simulink library "cpcAux"  (R2016a)
settings: Solver=ode45  StartTime=0.0  StopTime=10.0  RelTol=1e-3
undefined symbols (not defined in the file): DiscIntNeverNeededParam, sMP
libraries: simulink x16, cpcAux x8
(part 2 of 2)

== system cpcAux/cpcAux/Other/motion detected ==
  u : Inport
  Compare : RelationalOperator  Operator=>  OutDataTypeStr=fixdt(0, 8)  ZeroCross=off  InputSameDT=on
  Constant : Constant  DisableCoverage=on  Value=const  OutDataTypeStr=Inherit: Inherit via back propagation
  y : Outport
  wires:
  Compare/1 -> y/1
  Constant/1 -> Compare/2
  u/1 -> Compare/1

== system cpcAux/cpcAux/Shift/round for Voith DIWA transmissions ==
  note: round to defined resolution
  In1 : Inport
  Constant : Constant  Value=1/resolution
      settings: AttributesFormatString=%<Value>
  Divide : Product  Inputs=*/
  Product : Product
  Rounding Function : Rounding  Operator=round
  Out1 : Outport
  wires:
  In1/1 -> Product/1
  Divide/1 -> Out1/1
  Rounding Function/1 -> Divide/1
  Product/1 -> Rounding Function/1
  Constant/1 -> Product/2, Divide/2

== system cpcAux/cpcAux/Shift/shift manually for eActros ==
  kmh : Inport
  gear : Inport  Port=2
  sw_in : Inport  Port=3
  Chart : Stateflow chart  TreatAsAtomicUnit=on
  Constant : Constant  Value=bShiftManual
  SNA CurrGr : Subsystem  mask{sna_max=129, sna_eq=0}
      mask prompts: sna_max "max value"; sna_eq "equivalent value"
      mask help: If value above max value, it will be replaced by equivalent value
      settings: AttributesFormatString=x > %<sna_max>: %<sna_eq>
  consider manual shift from driver : Switch  Criteria=u2 > Threshold
  manual shift from cpcAux : Switch  Criteria=u2 > Threshold
  no shift : simulink/Logic and Bit Operations/Compare To Constant  relop===  const=1  OutDataTypeStr=boolean
  sw_out : Outport
  wires:
  manual shift from cpcAux/1 -> sw_out/1
  Constant/1 -> manual shift from cpcAux/2
  gear/1 -> SNA CurrGr/1(In)
  consider manual shift from driver/1 -> manual shift from cpcAux/1
  no shift/1 -> consider manual shift from driver/2
  Chart/1(sw) -> consider manual shift from driver/1
  kmh/1 -> Chart/1(kmh)
  sw_in/1 -> no shift/1, consider manual shift from driver/3, manual shift from cpcAux/3
  SNA CurrGr/1(Out) -> Chart/2(gear)

== system cpcAux/cpcAux/eActros Drivertrain ready/PT Ready Check ==
  PT_ready : Inport
  Enable : EnablePort
  Constant : Constant
  Discrete-Time Integrator : DiscreteIntegrator  gainval=1  InitialConditionSetting=State (most efficient)  SampleTime=-1  ICPrevOutput=DiscIntNeverNeededParam  ICPrevScaledInput=DiscIntNeverNeededParam
  Logical Operator : Logic  Operator=OR  AllPortsSameDT=off  OutDataTypeStr=boolean
  Logical Operator1 : Logic  Operator=NOT  Inputs=1  AllPortsSameDT=off  OutDataTypeStr=boolean
  Stop__Powertrain_not_ready : Stop  Description=The simulation completes the current time step before terminating
      settings: AttributesFormatString=%<Description>
  affter 1min : simulink/Logic and Bit Operations/Compare To Constant  relop=<  const=60  OutDataTypeStr=boolean
  error_pt_ready : Assertion  AssertionFailFcn=fprintf(2,'cpcAux: PT not ready, even after 60s after ignition\n')  StopWhenAssertionFail=off
  wires:
  Logical Operator1/1 -> Stop__Powertrain_not_ready/1
  Logical Operator/1 -> error_pt_ready/1, Logical Operator1/1
  affter 1min/1 -> Logical Operator/1
  Discrete-Time Integrator/1 -> affter 1min/1
  Constant/1 -> Discrete-Time Integrator/1
  PT_ready/1 -> Logical Operator/2

== system cpcAux/cpcAux/CruiseControl/CC controlled by IPPC/Interval ==
  u : Inport
  AND : Logic  AllPortsSameDT=off  OutDataTypeStr=boolean
  FixPt Data Type Duplicate : DataTypeDuplicate  DisableCoverage=on  NumInputPorts=3
  Lower Limit : Constant  DisableCoverage=on  Value=lowlimit  OutDataTypeStr=Inherit: Inherit via back propagation
  Lower Test : RelationalOperator  DisableCoverage=on  Operator=<=  OutDataTypeStr=boolean  ZeroCross=off
  Upper Limit : Constant  DisableCoverage=on  Value=uplimit  OutDataTypeStr=Inherit: Inherit via back propagation
  Upper Test : RelationalOperator  DisableCoverage=on  Operator=<=  OutDataTypeStr=boolean  ZeroCross=off
  y : Outport
  wires:
  AND/1 -> y/1
  u/1 -> Upper Test/1, Lower Test/2, FixPt Data Type Duplicate/1
  Upper Test/1 -> AND/2
  Lower Test/1 -> AND/1
  Upper Limit/1 -> FixPt Data Type Duplicate/3, Upper Test/2
  Lower Limit/1 -> FixPt Data Type Duplicate/2, Lower Test/1

== system cpcAux/cpcAux/CruiseControl/CC controlled by IPPC/Interval1 ==
  u : Inport
  AND : Logic  AllPortsSameDT=off  OutDataTypeStr=boolean
  FixPt Data Type Duplicate : DataTypeDuplicate  DisableCoverage=on  NumInputPorts=3
  Lower Limit : Constant  DisableCoverage=on  Value=lowlimit  OutDataTypeStr=Inherit: Inherit via back propagation
  Lower Test : RelationalOperator  DisableCoverage=on  Operator=<=  OutDataTypeStr=boolean  ZeroCross=off
  Upper Limit : Constant  DisableCoverage=on  Value=uplimit  OutDataTypeStr=Inherit: Inherit via back propagation
  Upper Test : RelationalOperator  DisableCoverage=on  Operator=<=  OutDataTypeStr=boolean  ZeroCross=off
  y : Outport
  wires:
  AND/1 -> y/1
  u/1 -> Upper Test/1, Lower Test/2, FixPt Data Type Duplicate/1
  Upper Test/1 -> AND/2
  Lower Test/1 -> AND/1
  Upper Limit/1 -> FixPt Data Type Duplicate/3, Upper Test/2
  Lower Limit/1 -> FixPt Data Type Duplicate/2, Lower Test/1

== system cpcAux/cpcAux/Ignition/calc IgnSw_Stat_SCA (moved to stateflow chart)/Interval ==
  u : Inport
  AND : Logic  AllPortsSameDT=off  OutDataTypeStr=boolean
  FixPt Data Type Duplicate : DataTypeDuplicate  DisableCoverage=on  NumInputPorts=3
  Lower Limit : Constant  DisableCoverage=on  Value=lowlimit  OutDataTypeStr=Inherit: Inherit via back propagation
  Lower Test : RelationalOperator  DisableCoverage=on  Operator=<=  OutDataTypeStr=boolean  ZeroCross=off
  Upper Limit : Constant  DisableCoverage=on  Value=uplimit  OutDataTypeStr=Inherit: Inherit via back propagation
  Upper Test : RelationalOperator  DisableCoverage=on  Operator=<=  OutDataTypeStr=boolean  ZeroCross=off
  y : Outport
  wires:
  AND/1 -> y/1
  u/1 -> Upper Test/1, Lower Test/2, FixPt Data Type Duplicate/1
  Upper Test/1 -> AND/2
  Lower Test/1 -> AND/1
  Upper Limit/1 -> FixPt Data Type Duplicate/3, Upper Test/2
  Lower Limit/1 -> FixPt Data Type Duplicate/2, Lower Test/1

== system cpcAux/cpcAux/Ignition/calc IgnSw_Stat_SCA (moved to stateflow chart)/Set_Reset_State ==
  S : Inport  PortDimensions=1
  R : Inport  Port=2  OutDataTypeStr=boolean  PortDimensions=1
  Logical Operator : Logic  Operator=OR  AllPortsSameDT=off  OutDataTypeStr=boolean
  Logical Operator1 : Logic  OutDataTypeStr=boolean
  Logical Operator2 : Logic  Operator=NOT  OutDataTypeStr=boolean
  Memory : Memory  InheritSampleTime=on
  Q : Outport  OutDataTypeStr=boolean  PortDimensions=1  InitialOutput=0
  wires:
  Memory/1 -> Logical Operator/1
  S/1 -> Logical Operator/2
  R/1 -> Logical Operator2/1
  Logical Operator/1 -> Logical Operator1/1
  Logical Operator2/1 -> Logical Operator1/2
  Logical Operator1/1 -> Q/1, Memory/1

== system cpcAux/cpcAux/Shift/shift manually for eActros/SNA CurrGr ==
  In : Inport
  Constant : Constant  Value=sna_eq
  Switch : Switch  Criteria=u2 > Threshold  Threshold=sna_max
  Out : Outport
  wires:
  Constant/1 -> Switch/1
  Switch/1 -> Out/1
  In/1 -> Switch/2, Switch/3

== stateflow chart cpcAux/Transfer Gear Box/transfer case state ==
  (default) -> (junction 34)
  (junction 34) -> (junction 66) [order 1] : [x_n~= 3 && ...
      |  x_id>=0] % x_id not used yet
  (junction 66) -> (junction 35) [order 1] : % VG2800 identified
      | [x_trqDistr(2) > 60 && x_trqDistr(2) < 90]
  (junction 35) -> (junction 44) : % 0=HIGH / onroad
      | % 1=LOW / offroad
      | % 2=NEUTRAL
      | {TrfGboxGear = x_n;}
  (junction 44) -> (junction 73)
  (junction 73) -> (junction 46) : % SNA
      | {FrontAxleEng = 3;}
  (junction 46) -> (junction 84) : % no condition
      | % tested
  (junction 84) -> (junction 86) : % Differential lock
      | % Interaxle central
      | % engaged assumed
      | {InterAxleDrfLock = 1;}
  (junction 66) -> (junction 70) [order 2]
  (junction 34) -> (junction 58) [order 2] : {
      | TrfGboxGear = 3; % SNA
      | FrontAxleEng = 3; % SNA
      | InterAxleDrfLock = 3; %SNA
      | }
  (junction 70) -> (junction 37) : % VG3000 assumed
  (junction 37) -> (junction 75) : {TrfGboxGear = 3;}
  (junction 75) -> (junction 76) [order 1] : [x_trqDistr(1) == 0]
  (junction 76) -> (junction 78) : % Front axle disengaged
      | {FrontAxleEng = 0;}
  (junction 75) -> (junction 104) [order 2]
  (junction 78) -> (junction 82)
  (junction 104) -> (junction 80)
  (junction 80) -> (junction 82) : % Front axle engaged
      | {FrontAxleEng = 1;}
  (junction 82) -> (junction 91)
  (junction 91) -> (junction 89) : % SNA
      | {InterAxleDrfLock = 3;}
  data: InterAxleDrfLock output double =3; FrontAxleEng output double =3; TrfGboxGear output double =3; x_trqDistr parameter; x_id parameter; x_n parameter

== stateflow chart cpcAux/Blinds/Blinds ==
  state blind
    state grill [parallel]
      settings: executionOrder=1
      state open
        entry: PosGrill = 0;
      state close
        entry: PosGrill = 1;
      (default) -> blind.grill.open
      blind.grill.open -> blind.grill.close : [ Pos1 > 0 && Pos1 < 10 ]
      blind.grill.close -> blind.grill.open : [ Pos1 == 0 ]
    state bumper [parallel]
      settings: executionOrder=2
      state open
        entry: PosBumper = 0;
      state close
        entry: PosBumper = 2;
      (default) -> blind.bumper.open
      blind.bumper.open -> blind.bumper.close : [ Pos2 > 0 && Pos2 < 10 ]
      blind.bumper.close -> blind.bumper.open : [ Pos2 == 0 ]
  (default) -> blind
  data: Pos1 input; Pos2 input; PosGrill output; PosBumper output

== stateflow chart cpcAux/Blinds/LIN ==
  state Loop
    entry:
    Pos1 = uint8(15); % SNA
    Pos2 = uint8(15); % SNA
    Loop -> (junction 95) : % BlindPos
    (junction 95) -> (junction 115) [order 1] : [ReqId == 0]
    (junction 95) -> (junction 108) [order 2]
    (junction 115) -> (junction 97) : {Pos1 = ReqPos;}
    (junction 108) -> (junction 116) [order 1] : [ReqId == 1]
    (junction 108) -> (junction 104) [order 2]
    (junction 116) -> (junction 107) : {Pos2 = ReqPos;}
    (junction 104) -> (junction 105) [order 1] : [ReqId == 2]
    (junction 104) -> (junction 98) [order 2] : % do nothing
    (junction 105) -> (junction 94) : {Pos1 = ReqPos;
        | Pos2 = ReqPos;}
    (junction 94) -> (junction 98)
    (junction 107) -> (junction 94)
    (junction 97) -> (junction 107)
    (junction 98) -> (junction 110)
  data: ReqId input; ReqPos input; Pos1 output uint8; Pos2 output uint8

== stateflow chart cpcAux/CruiseControl/cc_set_check/cc_set_check ==
  state different/
    en:
    T = t;
    v_set_last = v_set;
  state error/
    en:
    sta_err = true;
  state identical/
    en:
    sta_err = false;
  (junction 23) -> different : % v_set is not equal v_ref
      | % (with a tolerance of 0.3 km/h)
      | [abs(v_ref - v_set) > 0.3]
  identical -> (junction 23) : % CC active
      | [cc_flag && ~cc_off]
  different -> error [order 3] : % difference exists
      | % within delta_T
      | [t > T + 5]
  different -> (junction 16) [order 2]
  different -> (junction 19) [order 1]
  different -> (junction 51) [order 4]
  (junction 16) -> identical : % v_set is equal v_ref
      | % (with a tolerance of 0.3 km/h)
      | [abs(v_ref - v_set) <= 0.3]
  (junction 19) -> identical : % CC deactive
      | [~cc_flag || cc_off]
  (default) -> identical : % start
      | {sta_err = false;}
  (junction 51) -> identical : % CC inc or dec switch (not operated)
      | %  && v_set changes
      | [cc_spdChangeRq && v_set ~= v_set_last]
  data: t input double; v_ref input double; v_set input double; T local double; cc_flag input boolean; cc_off input boolean; sta_err output boolean; cc_spdChangeRq input boolean; v_set_last local double

== stateflow chart cpcAux/CruiseControl/cc_set_check/hyst_lower_check ==
  state different/
    en:
    T = t;
    v_hyst_last = v_hyst;
    v_hyst_ref_last = v_hyst_ref;
  state error/
    en:
    sta_err = true;
  state identical/
    en:
    sta_err = false;
  (junction 23) -> different : % drv change req
      | [v_hyst_ref ~= v_hyst]
  (junction 37) -> (junction 23) : % CC inc or dec switch
      | % not operated
      | [~cc_spdChangeRq]
  different -> (junction 30) [order 4] : % drv req has changed
      | [v_hyst_ref ~= v_hyst_ref_last]
  (junction 30) -> identical
  different -> error [order 6] : % no change of v_hyst
      | % within delta_T
      | [t > T + 5.0]
  identical -> (junction 37) : % CC active
      | [cc_flag && ~cc_off]
  different -> (junction 29) [order 3] : % v_hyst has changed
      | [v_hyst ~= v_hyst_last]
  (junction 29) -> identical
  different -> (junction 16) [order 2]
  different -> (junction 19) [order 1]
  different -> (junction 39) [order 5]
  (junction 16) -> identical : % drv req. equal v_hyst
      | [v_hyst_ref == v_hyst]
  (junction 19) -> identical : % CC deactive
      | [~cc_flag || cc_off]
  (default) -> identical : % start
      | {sta_err = false;}
  (junction 39) -> identical : % CC inc or dec switch
      | % operated
      | [cc_spdChangeRq]
  data: t input double; v_hyst_ref input double; v_hyst input double; v_hyst_last local double; T local double; cc_flag input boolean; cc_off input boolean; sta_err output boolean; v_hyst_ref_last local double; cc_spdChangeRq input boolean

== stateflow chart cpcAux/CruiseControl/cc_set_check/hyst_upper_check ==
  state different/
    en:
    T = t;
    v_hyst_last = v_hyst;
    v_hyst_ref_last = v_hyst_ref;
  state error/
    en:
    sta_err = true;
  state identical/
    en:
    sta_err = false;
  (junction 23) -> different : % drv change req
      | [v_hyst_ref ~= v_hyst]
  (junction 37) -> (junction 23) : % CC inc or dec switch
      | % not operated
      | [~cc_spdChangeRq]
  different -> (junction 30) [order 4] : % drv req has changed
      | [v_hyst_ref ~= v_hyst_ref_last]
  (junction 30) -> identical
  different -> error [order 6] : % no change of v_hyst
      | % within delta_T
      | [t > T + 5.0]
  identical -> (junction 37) : % CC active
      | [cc_flag && ~cc_off]
  different -> (junction 29) [order 3] : % v_hyst has changed
      | [v_hyst ~= v_hyst_last]
  (junction 29) -> identical
  different -> (junction 16) [order 2]
  different -> (junction 19) [order 1]
  different -> (junction 39) [order 5]
  (junction 16) -> identical : % drv req. equal v_hyst
      | [v_hyst_ref == v_hyst]
  (junction 19) -> identical : % CC deactive
      | [~cc_flag || cc_off]
  (default) -> identical : % start
      | {sta_err = false;}
  (junction 39) -> identical : % CC inc or dec switch
      | % operated
      | [cc_spdChangeRq]
  data: t input double; v_hyst_ref input double; v_hyst input double; v_hyst_last local double; T local double; cc_flag input boolean; cc_off input boolean; sta_err output boolean; v_hyst_ref_last local double; cc_spdChangeRq input boolean

== stateflow chart cpcAux/CruiseControl/cc ==
  state Pause_Speed
    en:
    T = t;
    cc_spd_inc_sw = 0;
    cc_spd_dec_sw = 0;
    cc_lohyst_inc_sw = 0;
    cc_lohyst_dec_sw = 0;
    cc_uphyst_inc_sw = 0;
    cc_uphyst_dec_sw = 0;
  state cc_init
    en:
    v_set_init = 0;
    T = t;
    cc_spd_inc_sw = 0;
    cc_spd_dec_sw = 0;
    cc_lohyst_inc_sw = 0;
    cc_lohyst_dec_sw = 0;
    cc_uphyst_inc_sw = 0;
    cc_uphyst_dec_sw = 0;
    cc_mode_a_sw = 0;
  state Run
    en:
    v_set_init = v_set;
    cc_spd_inc_sw = 0;
    cc_spd_dec_sw = 0;
    cc_lohyst_inc_sw = 0;
    cc_lohyst_dec_sw = 0;
    cc_uphyst_inc_sw = 0;
    cc_uphyst_dec_sw = 0;
    cc_mode_a_sw = 0;
  state Pause_ACCP
    en:
    T = t;
    cc_spd_dec_sw = 0;
  state Inc_SetSpeed
    en:
    T = t;
    cc_spd_inc_sw = 1;
  state Inc_HoldPos
  state Resume_ACCP
    en:
    T = t;
    cc_spd_dec_sw = 1;
  state Dec_SetSpeed
    en:
    T = t;
    cc_spd_dec_sw = 1;
  state Dec_HoldPos
  state Deactivate_CC
    en:
    T = t;
    cc_off_sw = 1;
    exit:
    cc_off_sw = 0;
  state Inc_UpperHyst
    en:
    T = t;
    cc_uphyst_inc_sw = 1;
  state Change_CC_Mode
    // 0 = none (OK)
    // 1 = Road Speed Limiter (OK)
    // 2 = Combined (OK)
    // 3 = Drive CC (OK)
    // 4 = Adaptive CC (OK)
    // 5 = Adaptive CC+ (OK)
    // 6..13 = Reserved (OOR)
    // 14 = error (ERR)
    // 15 = sna (SNA)
    en:
    T = t;
    cc_mode_a_sw = 1;
  state Wait_for_Activate_CC
  state Activate_CC
    en:
    T = t;
    cc_spd_inc_sw = 1;
  state Dec_UpperHyst
    en:
    T = t;
    cc_uphyst_dec_sw = 1;
  state Wait_CC
    en:
    T = t;
    cc_spd_inc_sw = 0;
    cc_spd_dec_sw = 0;
  state Inc_LowerHyst
    en:
    T = t;
    cc_lohyst_inc_sw = 1;
  state Resume_CC
    en:
    T = t;
    cc_spd_dec_sw = 1;
  state Dec_LowerHyst
    en:
    T = t;
    cc_lohyst_dec_sw = 1;
  state Pause_CC_Mode
    en:
    T = t;
    cc_mode_a_sw = 0;
  (default) -> cc_init
  Pause_Speed -> (junction 71) : [t > T+0.1]
  (junction 71) -> Run
  (junction 286) -> Pause_Speed : [t > T+0.1]
      | // short tick
  Pause_ACCP -> Run : [t > T + 1.0]
  Inc_SetSpeed -> Inc_HoldPos [order 4] : [v_set_ref - v_set >= 2.5 && ...
      |  (v_set_ref %% 10==0 || v_set_ref %% 5==0)]
  Run -> Inc_SetSpeed [order 4] : [(v_set < v_set_ref-0.3) && ...
      | ippc_setspd_ctrl==0]
  Inc_SetSpeed -> Inc_HoldPos [order 3] : [v_set_ref - v_set >= 5]
  Resume_ACCP -> Pause_ACCP : [t > T+0.1]
  Inc_SetSpeed -> Run [order 2] : [v_set_ref - v_set <= 0]
  Inc_HoldPos -> Inc_SetSpeed : [t>T+0.5] // long tick
  Inc_SetSpeed -> (junction 286) [order 5]
  Inc_SetSpeed -> Run [order 1] : [cc_flag == 0 || cc_off == 1] // CC deactivation
  (junction 335) -> (junction 286)
  Run -> Resume_ACCP [order 3] : [v_v < 0.5 && ...
      | acc_drive_rdy == 1]
  Dec_SetSpeed -> Dec_HoldPos [order 4] : [v_set_ref - v_set <= -2.5 && ...
      |  (v_set_ref %% 10==0 || v_set_ref %% 5==0)]
  Run -> Dec_SetSpeed [order 5] : [(v_set > v_set_ref+0.3) && ...
      | ippc_setspd_ctrl==0]
  cc_init -> (junction 353) : [ready2drive == 1]
  Dec_SetSpeed -> Dec_HoldPos [order 3] : [v_set_ref - v_set <= -5]
  Dec_SetSpeed -> Run [order 2] : [v_set_ref - v_set >= 0]
  Dec_HoldPos -> Dec_SetSpeed : [t>T+0.5] // long tick
  Deactivate_CC -> (junction 181) : [t > T + 0.1]
  Dec_SetSpeed -> Run [order 1] : [cc_flag == 0 || cc_off == 1] // CC deactivation
  Dec_SetSpeed -> (junction 335) [order 5]
  Run -> Deactivate_CC [order 2] : [cc_flag == 0] // CC deactivation command by driver
  (junction 181) -> Wait_for_Activate_CC
  (junction 342) -> (junction 335)
  (junction 353) -> (junction 137) : [t > T+0.1]
  Run -> Wait_for_Activate_CC [order 1] : [cc_off == 1] // CC is deactivated for some reason
  Run -> Inc_UpperHyst [order 6] : [v_hyst_upper < v_hyst_upper_ref-0.3]
  Inc_UpperHyst -> (junction 306)
  (junction 306) -> (junction 342)
  (junction 308) -> (junction 306)
  (junction 137) -> Change_CC_Mode [order 2]
  (junction 137) -> Wait_for_Activate_CC [order 1] : [cc_fun_z == CCFunc]
  Activate_CC -> Run [order 1] : [t > T+0.1 && ...
      | cc_off == 0]
  Pause_CC_Mode -> (junction 137) : [t > T+0.1]
  Wait_for_Activate_CC -> Activate_CC [order 2] : [cc_flag == 1]
  Run -> Dec_UpperHyst [order 7] : [v_hyst_upper > v_hyst_upper_ref+0.3]
  Dec_UpperHyst -> (junction 308)
  Activate_CC -> Wait_CC [order 2] : [t > T+0.1 && ...
      | cc_off == 1]
  (junction 307) -> (junction 308)
  Wait_CC -> Wait_for_Activate_CC [order 2] : [t > T+1.0 && ...
      | cc_off == 1]
  Wait_CC -> Run [order 1] : [cc_off == 0]
  Inc_LowerHyst -> (junction 307)
  Run -> Inc_LowerHyst [order 8] : [v_hyst_lower < v_hyst_lower_ref-0.3]
  Wait_for_Activate_CC -> Resume_CC [order 1] : [cc_flag == 1 && ...
      | v_set_init > 0 && ...
      | (abs(v_set_ref - v_set_init) < ...
      | abs(v_set_ref - v_v))]
  (junction 309) -> (junction 307)
  Change_CC_Mode -> Pause_CC_Mode : [t > T+0.1]
  Resume_CC -> Wait_CC [order 2] : [t > T+0.1 && ...
      | cc_off == 1]
  Resume_CC -> Run [order 1] : [t > T+0.1 && ...
      | cc_off == 0]
  Dec_LowerHyst -> (junction 309)
  Run -> Dec_LowerHyst [order 9] : [v_hyst_lower > v_hyst_lower_ref+0.3]
  data: t input double; cc_uphyst_inc_sw output uint8; cc_uphyst_dec_sw output uint8; cc_lohyst_inc_sw output uint8; cc_lohyst_dec_sw output uint8; ready2drive input int8; cc_spd_inc_sw output uint8; cc_mode_a_sw output uint8; cc_spd_dec_sw output uint8; cc_off_sw output uint8 =0; v_v input double; v_set_ref input double; cc_flag input uint8; v_hyst_lower_ref input double; v_hyst_upper_ref input double; cc_off input uint8; T local double; v_set input double; v_hyst_lower input double; v_hyst_upper input double; cc_fun_z input uint8; acc_drive_rdy input uint8; v_set_init local double; ippc_setspd_ctrl input boolean; CCFunc parameter

== stateflow chart cpcAux/Ignition/ignition status  ==
  state Ignition_Off
    en:
    ign_rdy = 0;
    ign_z = 0;
  state Ignition_Accessory_15R
    en:
    ign_z = 1;
  state Ignition_On_15
    en:
    ign_z = 2;
  state ShiftPrg
  state Ignition_Crank_50
    en:
    ign_z = 3;
  state Ignition_after_Crank
    en:
    ign_z = 2;
    ign_rdy = 1;
  (default) -> Ignition_Off
  Ignition_Off -> Ignition_Accessory_15R : % Should be usually after 0.1s
      | [drv_ign == 1]
  Ignition_Accessory_15R -> Ignition_On_15 : after(0.1, sec)
  Ignition_On_15 -> ShiftPrg [order 1] : /* Shift Program selected
      | (AgModulState ~= 1)*/
      | [ShiftPrg < 255]
  Ignition_On_15 -> Ignition_Crank_50 [order 2] : /* fallback
      | solution */
      | after(5, sec)
  ShiftPrg -> Ignition_Crank_50 [order 1] : /* conventional
      | (EngSpd not SNA) */
      | [EngSpd <= 8000]
  ShiftPrg -> Ignition_Crank_50 [order 2] : /* electric */
      | [HvRdy == 1]
  ShiftPrg -> Ignition_Crank_50 [order 3] : /* fallback
      | solution */
      | after(5, sec)
  Ignition_Crank_50 -> Ignition_after_Crank [order 1] : /* conventional */
      | [EngSpd > 450 ...
      | && EngSpd <= 8000]
  Ignition_Crank_50 -> Ignition_after_Crank [order 2] : /* fallback solution
      | (also for electric) */
      | after(1.2, sec)
  data: ign_z output uint8; ign_rdy output boolean; drv_ign input uint8; ShiftPrg input uint8; HvRdy input boolean; EngSpd input

== stateflow chart cpcAux/Shift/drive mode switch ==
  state Init
    en:
    init_sta = 1; // init ongoing
    mode_rq = 1; // Drive (D)
    AutoManSw = 0;
    ready2drive = 0;
    prg_count = 0;
  state Switch_D_N_R
    // N = 1
    // D = 2
    // R = 4
    en: mode_rq = drv_RND;
  state Error_M
    /* Vehicle stays
    in automatic */
    en: ready2drive = -1;
  state Switch_M
    en: AutoManSw = 1;
  state SftPrg
    // Change Driving Program
    en: AutoManSw = 1;
    ex: AutoManSw = 0;
  state SftPrg_Changed
    /* Drive Program changed to next one
    and iIncrease program change counter */
    en: prg_count += 1;
  state Error_Prg
    /* Could not switch into requested
    drive program after 2nd attempt,
    but CPC only support 3 drive prog. */
    en: ready2drive = -2;
  state Ready2Drive
    en:
    init_sta = 0;
    ready2drive = 1;
    AutoManSw = 0;
  state Driving_AT
    // Automatic Transmission
  state Driving_AMT
    // Auto. Manual Transm.
    /* Driver can change mode
    for coasting for example */
    du: mode_rq = drv_RND;
  state Neutral_by_Veh
    /* Switch to Neutral (N),
    to be able to engage gear
    by Drive (D) again */
    en: mode_rq = 1;
    ex: mode_rq = drv_RND;
  (default) -> Init
  Init -> Switch_D_N_R : [rdy == 1]
  Switch_D_N_R -> (junction 413) [order 1] : /* Do not wait for
      | AT transmission */
      | [tcm_SysID== 2 ...
      | || tcm_SysID == 10]
  Switch_D_N_R -> (junction 415) [order 2] : /* Wait for TCM
      | to engage a gear */
      | [mode_rq == 2 ... D
      | && gear > 0 ...
      | && gear < 130]
  Switch_D_N_R -> (junction 416) [order 3] : // Gear in neutral
      | [mode_rq == 1 ... N
      | && gear == 0]
  (junction 413) -> (junction 415)
  (junction 415) -> (junction 416)
  (junction 416) -> (junction 366)
  Switch_M -> Error_M [order 2] : after(1, sec)
  (junction 392) -> SftPrg : /* Drive Program
      | not selected by CPC */
      | [ShiftPrg ~= prg]
  (junction 366) -> (junction 392) [order 2] : /* Explicit Drive Program
      | defined */
      | [ShiftPrg ~= 255]
  (junction 406) -> Switch_M [order 1] : // In automatic
      | [AutoManDisp == 1]
  (junction 366) -> (junction 406) [order 1] : // Manaul Shift defined
      | [bShiftManual == 1]
  (junction 406) -> (junction 408) [order 2]
  (junction 366) -> (junction 395) [order 3]
  SftPrg -> SftPrg_Changed : after(0.1, sec)
  SftPrg_Changed -> SftPrg [order 3] : /* Wait to change
      | Driving Program again */
      | after(1,sec)
  Switch_M -> (junction 369) [order 1] : // Not in automatic
      | // SNA also accepted
      | [after(0.5, sec) ...
      | && AutoManDisp ~= 1]
  (junction 369) -> (junction 408)
  (junction 408) -> (junction 395)
  SftPrg_Changed -> (junction 395) [order 1] : /* Drive Program
      | selected by CPC */
      | [ShiftPrg == prg]
  (junction 395) -> Ready2Drive
  SftPrg_Changed -> Error_Prg [order 2] : [prg_count >= 2]
  Ready2Drive -> (junction 433)
  (junction 433) -> Driving_AT [order 1] : [tcm_SysID== 2 ...
      | || tcm_SysID == 10]
  (junction 433) -> (junction 424) [order 2]
  Neutral_by_Veh -> Driving_AMT : after(1, sec)
  (junction 424) -> Driving_AMT
  Driving_AMT -> Neutral_by_Veh : // Check, if vehicle goes to neutral at stop
      | after(1, sec) [drv_RND== 2 && gear == 0 && speed < 0.1]
  data: rdy input boolean; AutoManDisp input double; tcm_SysID input double; gear input double; init_sta output boolean; mode_rq output uint8; speed input double; AutoManSw output uint8; ready2drive output int8; bShiftManual parameter; ShiftPrg parameter; prg_count local uint8; prg input double; drv_RND input double

== stateflow chart cpcAux/Shift/shift manually for eActros/Chart ==
  state Downshift
    en: sw = 2;
  state NoShift
    en: sw = 1;
  state Upshift
    en: sw = 4;
  state Wait
    en: sw = 1;
  (default) -> NoShift
  NoShift -> Upshift [order 1] : [gear ~=0 && kmh > kmh_upshift(gear)]
  NoShift -> Downshift [order 2] : [gear ~=0 && kmh < kmh_downshift(gear)]
  Downshift -> (junction 15) : after(0.2, sec)
  Wait -> NoShift : after(s_shift_wait, sec)
  Upshift -> (junction 18) : after (0.2, sec)
  (junction 15) -> Wait
  (junction 18) -> Wait
  data: sw output; kmh input; gear input; kmh_upshift parameter; kmh_downshift parameter; s_shift_wait parameter
